simulink model "train_system"  (R2022b)
settings: Solver=VariableStepAuto  StartTime=0.0  StopTime=1000  MaxStep=0.01  RelTol=1e-3
undefined symbols (not defined in the file or in its folder): g, k, M1, M2, mu
settings Model: Creator=Brigosha_Guest  LastModifiedBy=Brigosha_Guest

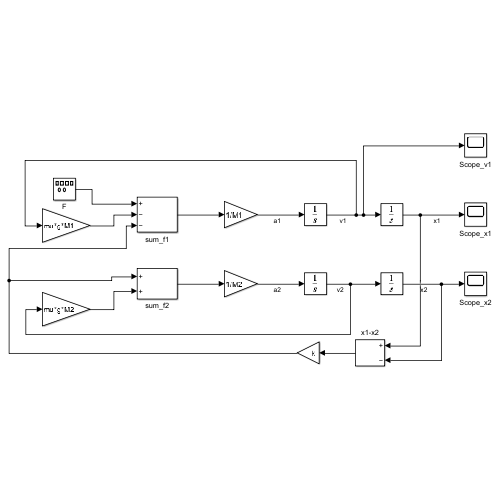
[thumbnail: Simulink's stored preview of the top-level diagram]
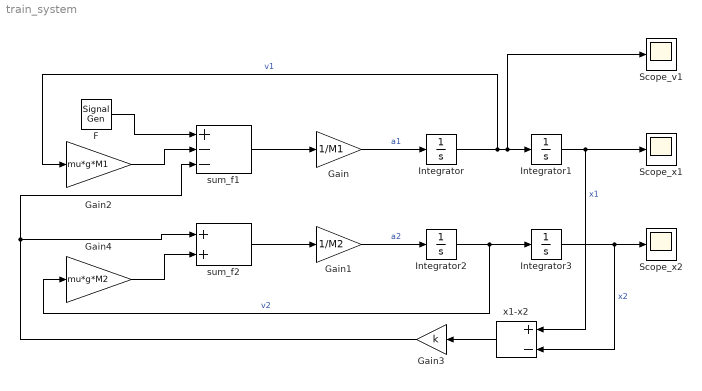
== system train_system ==
  F : SignalGenerator  WaveForm=square  Amplitude=-1  Frequency=0.001
  Gain : Gain  Gain=1/M1
  Gain1 : Gain  Gain=1/M2
  Gain2 : Gain  Gain=mu*g*M1
  Gain3 : Gain  Gain=k
  Gain4 : Gain  Gain=mu*g*M2
  Integrator{,1..3} (4 alike) : Integrator
  Scope_v1 : Scope
  Scope_x1 : Scope
  Scope_x2 : Scope
  sum_f1 : Sum  Inputs=+--
  sum_f2 : Sum
  x1-x2 : Sum  Inputs=+-
  wires:
  sum_f1/1 -> Gain/1
  sum_f2/1 -> Gain1/1
  Gain/1 -> Integrator/1  "a1"
  Integrator/1 -> Gain2/1, Scope_v1/1, Integrator1/1  "v1"
  Integrator2/1 -> Gain4/1, Integrator3/1  "v2"
  Gain1/1 -> Integrator2/1  "a2"
  Integrator1/1 -> x1-x2/1, Scope_x1/1  "x1"
  Integrator3/1 -> x1-x2/2, Scope_x2/1  "x2"
  F/1 -> sum_f1/1
  Gain2/1 -> sum_f1/2
  x1-x2/1 -> Gain3/1
  Gain3/1 -> sum_f2/1, sum_f1/3
  Gain4/1 -> sum_f2/2
